simulink model "sim_mobile_robot_trajectory_control_pi"  (R2020b)
settings: Solver=ode1  StartTime=0.0  StopTime=100  FixedStep=0.01  RelTol=1e-3
libraries: pid_lib x2, simulink x2, dspsigops x1
settings Model: Creator=ONLY-GOD  LastModifiedBy=ONLY-GOD

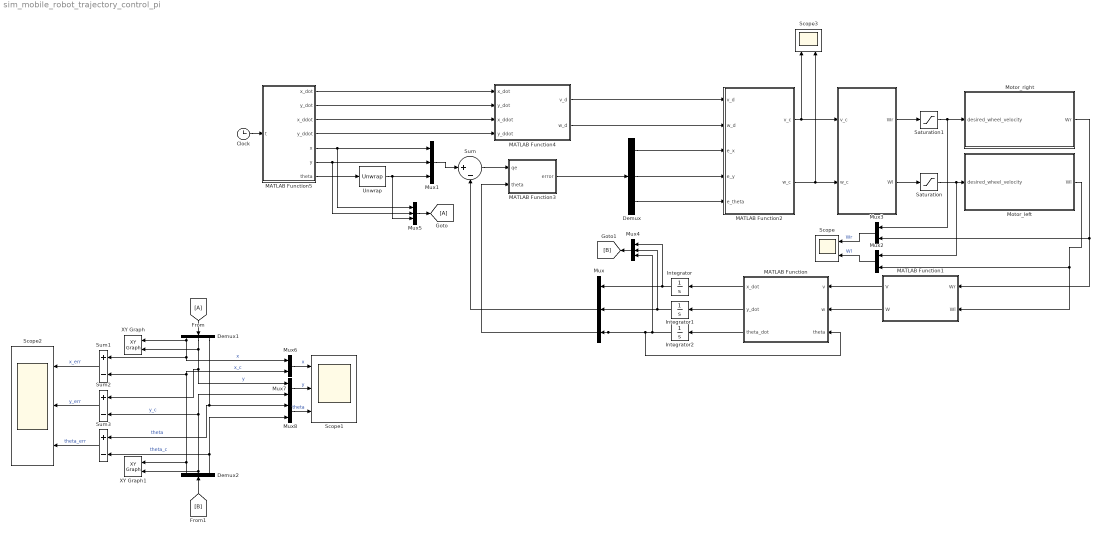
== system sim_mobile_robot_trajectory_control_pi ==
  " " : MATLAB Function  TreatAsAtomicUnit=on
  Clock : Clock
  Demux : Demux  Outputs=3
  Demux1 : Demux  Outputs=3
  Demux2 : Demux  Outputs=3
  Integrator : Integrator
  Integrator1 : Integrator
  Integrator2 : Integrator
  MATLAB Function : MATLAB Function  TreatAsAtomicUnit=on
  MATLAB Function1 : MATLAB Function  TreatAsAtomicUnit=on
  MATLAB Function2 : MATLAB Function  TreatAsAtomicUnit=on
  MATLAB Function3 : MATLAB Function  TreatAsAtomicUnit=on
  MATLAB Function4 : MATLAB Function  TreatAsAtomicUnit=on
  MATLAB Function5 : MATLAB Function  TreatAsAtomicUnit=on
  Motor_left : Subsystem
  Motor_right : Subsystem
  Mux{,1,4..5} (4 alike) : Mux  Inputs=3
  Mux{2..3,6..8} (5 alike) : Mux  Inputs=2
  Saturation : Saturate  UpperLimit=14  LowerLimit=-14
  Saturation1 : Saturate  UpperLimit=14  LowerLimit=-14
  Scope : Scope  NumInputPorts=2
  Scope1 : Scope  NumInputPorts=3
  Scope2 : Scope  NumInputPorts=3
  Scope3 : Scope  NumInputPorts=2
  Sum : Sum  Inputs=|+-
  Sum1 : Sum  Inputs=+-
  Sum2 : Sum  Inputs=+-
  Sum3 : Sum  Inputs=+-
  Unwrap : dspsigops/Unwrap  tol=pi  InputProcessing=Columns as channels (frame based)  running=off
  XY Graph : simulink/Sinks/XY Graph  xmin=-6  xmax=6  ymin=-6  ymax=6  st=-1
  XY Graph1 : simulink/Sinks/XY Graph  xmin=-6  xmax=6  ymin=-6  ymax=6  st=-1
  wires:
  Demux/1 -> MATLAB Function2/3(e_x)
  Demux/2 -> MATLAB Function2/4(e_y)
  Demux/3 -> MATLAB Function2/5(e_theta)
  Sum/1 -> MATLAB Function3/1(qe)
  MATLAB Function3/1(error) -> Demux/1
  MATLAB Function4/1(v_d) -> MATLAB Function2/1(v_d)
  MATLAB Function4/2(w_d) -> MATLAB Function2/2(w_d)
  MATLAB Function2/1(v_c) -> " "/1(v_c), Scope3/1
  MATLAB Function2/2(w_c) -> Scope3/2, " "/2(w_c)
  " "/1(Wr) -> Saturation1/1
  " "/2(Wl) -> Saturation/1
  Motor_right/1(Wr) -> Mux3/2, MATLAB Function1/1(Wr)
  Motor_left/1(Wl) -> Mux2/2, MATLAB Function1/2(Wl)
  MATLAB Function1/1(V) -> MATLAB Function/1(v)
  MATLAB Function1/2(W) -> MATLAB Function/2(w)
  MATLAB Function/3(theta_dot) -> Integrator2/1
  MATLAB Function/1(x_dot) -> Integrator/1
  MATLAB Function/2(y_dot) -> Integrator1/1
  Integrator2/1 -> Mux4/3, MATLAB Function3/2(theta), Mux/3, MATLAB Function/3(theta)
  Integrator/1 -> Mux4/1, Mux/1
  Integrator1/1 -> Mux4/2, Mux/2
  Mux/1 -> Sum/2
  MATLAB Function5/1(x_dot) -> MATLAB Function4/1(x_dot)
  MATLAB Function5/2(y_dot) -> MATLAB Function4/2(y_dot)
  MATLAB Function5/3(x_ddot) -> MATLAB Function4/3(x_ddot)
  MATLAB Function5/4(y_ddot) -> MATLAB Function4/4(y_ddot)
  Clock/1 -> MATLAB Function5/1(t)
  MATLAB Function5/5(x) -> Mux1/1, Mux5/1
  MATLAB Function5/6(y) -> Mux1/2, Mux5/2
  MATLAB Function5/7(theta) -> Unwrap/1
  Mux1/1 -> Sum/1
  Mux3/1 -> Scope/1  "Wr"
  Mux2/1 -> Scope/2  "Wl"
  Mux5/1 -> [A]
  Mux4/1 -> [B]
  [A] -> Demux1/1
  [B] -> Demux2/1
  Demux1/1 -> Mux6/1, Sum1/1, XY Graph/1  "x"
  Demux2/1 -> Mux6/2, Sum1/2, XY Graph1/1  "x_c"
  Demux1/2 -> Sum2/1, Mux7/1, XY Graph/2  "y"
  Demux2/2 -> Mux7/2, Sum2/2, XY Graph1/2  "y_c"
  Demux2/3 -> Mux8/2, Sum3/2  "theta_c"
  Mux6/1 -> Scope1/1  "x"
  Mux7/1 -> Scope1/2  "y"
  Mux8/1 -> Scope1/3  "theta"
  Demux1/3 -> Sum3/1, Mux8/1  "theta"
  Sum1/1 -> Scope2/1  "x_err"
  Sum2/1 -> Scope2/2  "y_err"
  Saturation1/1 -> Mux3/1, Motor_right/1(desired_wheel_velocity)
  Saturation/1 -> Mux2/1, Motor_left/1(desired_wheel_velocity)
  Unwrap/1 -> Mux5/3, Mux1/3
  Sum3/1 -> Scope2/3  "theta_err"

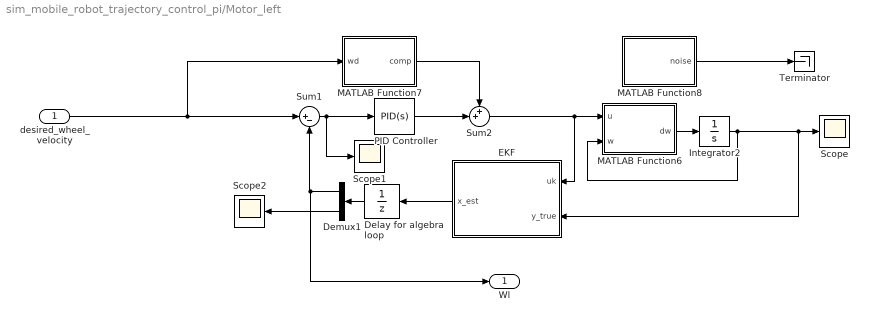
== system sim_mobile_robot_trajectory_control_pi/Motor_left ==
  desired_wheel_velocity : Inport
  Delay for algebra loop : UnitDelay  SampleTime=-1  HasFrameUpgradeWarning=on
  Demux1 : Demux  Outputs=[1,3]
  EKF : MATLAB Function  TreatAsAtomicUnit=on
  Integrator2 : Integrator
  MATLAB Function6 : MATLAB Function  TreatAsAtomicUnit=on
  MATLAB Function7 : MATLAB Function  TreatAsAtomicUnit=on
  MATLAB Function8 : MATLAB Function  TreatAsAtomicUnit=on
  PID Controller : pid_lib/PID Controller  Controller=PID  Form=Parallel  TimeDomain=Continuous-time  UseExternalTs=off  SampleTime=-1  IntegratorMethod=Forward Euler  FilterMethod=Forward Euler  ControllerParametersSource=internal  P=3*(27.65*(-1+2*1.5-2*sqrt(1.5*(1.5-1)))/17.35)  I=3*(27.65*(-1+2*1.5-2*sqrt(1.5*(1.5-1)))/17.35)* 1.5*27.65  D=0  UseFilter=on  N=100  TunerSelectOption=Transfer Function Based (PID Tuner App)  InitialConditionSource=internal  InitialConditionForIntegrator=0  InitialConditionForFilter=0  DifferentiatorICPrevScaledInput=0  ExternalReset=none  TrackingMode=off  Kt=1  LimitOutput=off  SatLimitsSource=internal  UpperSaturationLimit=inf  LowerSaturationLimit=-inf  LinearizeAsGain=on  AntiWindupMode=none  Kb=1  POutMin=[]  POutMax=[]  IOutMin=[]  IOutMax=[]  DOutMin=[]  DOutMax=[]  NOutMin=[]  NOutMax=[]  SumOutMin=[]  SumOutMax=[]  SaturationOutMin=[]  SaturationOutMax=[]  PParamMin=[]  PParamMax=[]  IParamMin=[]  IParamMax=[]  DParamMin=[]  DParamMax=[]  NParamMin=[]  NParamMax=[]  KbParamMin=[]  KbParamMax=[]  KtParamMin=[]  KtParamMax=[]  KbOutMin=[]  KbOutMax=[]  KtOutMin=[]  KtOutMax=[]  IntegratorOutMin=[]  IntegratorOutMax=[]  FilterOutMin=[]  FilterOutMax=[]  SumI1OutMin=[]  SumI1OutMax=[]  SumI2OutMin=[]  SumI2OutMax=[]  SumI3OutMin=[]  SumI3OutMax=[]  SumI4OutMin=[]  SumI4OutMax=[]  SumDOutMin=[]  SumDOutMax=[]  DifferentiatorOutMin=[]  DifferentiatorOutMax=[]  FilterDiffOutCoefMin=[]  FilterDiffOutCoefMax=[]  ReciprocalOutMin=[]  ReciprocalOutMax=[]  SumDenOutMin=[]  SumDenOutMax=[]  SumNumOutMin=[]  SumNumOutMax=[]  DivideOutMin=[]  DivideOutMax=[]  UdiffTsProdOutMin=[]  UdiffTsProdOutMax=[]  NTsProdOutMin=[]  NTsProdOutMax=[]  UintegralTsProdOutMin=[]  UintegralTsProdOutMax=[]  UngainTsProdOutMin=[]  UngainTsProdOutMax=[]  IntegratorContinuousStateAttributes=''  IntegratorStateMustResolveToSignalObject=off  IntegratorRTWStateStorageClass=Auto  FilterContinuousStateAttributes=''  FilterStateMustResolveToSignalObject=off  FilterRTWStateStorageClass=Auto  ParallelPVariant=InternalParameters  IdealPVariant=Disabled  IVariant=InternalParameters  DVariant=InternalParameters  IntegratorVariant=Continuous  SatVariant=Disabled  AWVariant=Passthrough  PCopyVariant=Disabled  TRVariant=Disabled  FdbkBlocksVariant=Forward  IdealPFdbkVariant=Disabled  SatFdbkVariant=Disabled  DerivativeFilterVariant=ContFilter  NVariant=InternalParameters  NCopyVariant=Disabled  FilterICVariant=InternalICsFilter  IntegratorICVariant=InternalICs  ExternalResetVariant=Disabled  TRSumVariant=Passthrough  SumFdbkVariant=Disabled  SumVariant=Sum_PID  TsampFilterVariant=InternalTs  TsampNgainVariant=Passthrough  TsampIntegralVariant=Passthrough  ExternalSaturationOutDataTypeStr=Inherit: Same as second input
  Scope : Scope
  Scope1 : Scope
  Scope2 : Scope
  Sum1 : Sum  Inputs=|+-
  Sum2 : Sum  Inputs=++|
  Terminator : Terminator
  Wl : Outport
  wires:
  Delay for algebra loop/1 -> Demux1/1
  Demux1/1 -> Wl/1, Sum1/2
  Integrator2/1 -> MATLAB Function6/2(w), Scope/1, EKF/2(y_true)
  MATLAB Function7/1(comp) -> Sum2/1
  Demux1/2 -> Scope2/1
  MATLAB Function8/1(noise) -> Terminator/1
  EKF/1(x_est) -> Delay for algebra loop/1
  MATLAB Function6/1(dw) -> Integrator2/1
  PID Controller/1 -> Sum2/2
  Sum1/1 -> PID Controller/1, Scope1/1
  desired_wheel_velocity/1 -> Sum1/1, MATLAB Function7/1(wd)
  Sum2/1 -> MATLAB Function6/1(u), EKF/1(uk)

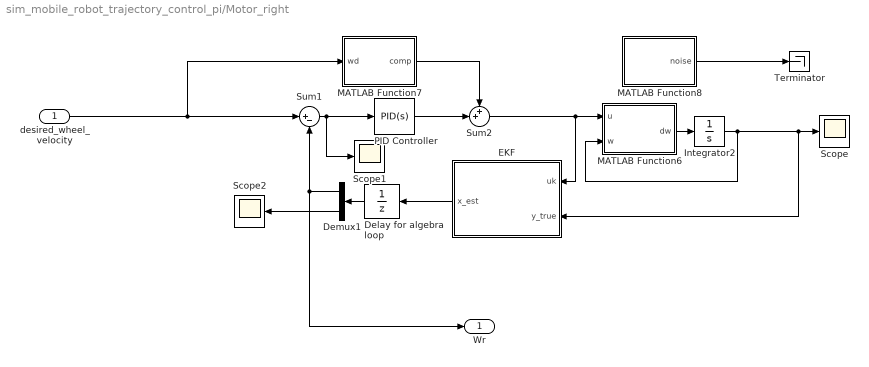
== system sim_mobile_robot_trajectory_control_pi/Motor_right ==
  desired_wheel_velocity : Inport
  Delay for algebra loop : UnitDelay  SampleTime=-1  HasFrameUpgradeWarning=on
  Demux1 : Demux  Outputs=[1,3]
  EKF : MATLAB Function  TreatAsAtomicUnit=on
  Integrator2 : Integrator
  MATLAB Function6 : MATLAB Function  TreatAsAtomicUnit=on
  MATLAB Function7 : MATLAB Function  TreatAsAtomicUnit=on
  MATLAB Function8 : MATLAB Function  TreatAsAtomicUnit=on
  PID Controller : pid_lib/PID Controller  Controller=PID  Form=Parallel  TimeDomain=Continuous-time  UseExternalTs=off  SampleTime=-1  IntegratorMethod=Forward Euler  FilterMethod=Forward Euler  ControllerParametersSource=internal  P=3*(27.65*(-1+2*1.5-2*sqrt(1.5*(1.5-1)))/17.35)  I=3*(27.65*(-1+2*1.5-2*sqrt(1.5*(1.5-1)))/17.35)* 1.5*27.65  D=0  UseFilter=on  N=100  TunerSelectOption=Transfer Function Based (PID Tuner App)  InitialConditionSource=internal  InitialConditionForIntegrator=0  InitialConditionForFilter=0  DifferentiatorICPrevScaledInput=0  ExternalReset=none  TrackingMode=off  Kt=1  LimitOutput=off  SatLimitsSource=internal  UpperSaturationLimit=inf  LowerSaturationLimit=-inf  LinearizeAsGain=on  AntiWindupMode=none  Kb=1  POutMin=[]  POutMax=[]  IOutMin=[]  IOutMax=[]  DOutMin=[]  DOutMax=[]  NOutMin=[]  NOutMax=[]  SumOutMin=[]  SumOutMax=[]  SaturationOutMin=[]  SaturationOutMax=[]  PParamMin=[]  PParamMax=[]  IParamMin=[]  IParamMax=[]  DParamMin=[]  DParamMax=[]  NParamMin=[]  NParamMax=[]  KbParamMin=[]  KbParamMax=[]  KtParamMin=[]  KtParamMax=[]  KbOutMin=[]  KbOutMax=[]  KtOutMin=[]  KtOutMax=[]  IntegratorOutMin=[]  IntegratorOutMax=[]  FilterOutMin=[]  FilterOutMax=[]  SumI1OutMin=[]  SumI1OutMax=[]  SumI2OutMin=[]  SumI2OutMax=[]  SumI3OutMin=[]  SumI3OutMax=[]  SumI4OutMin=[]  SumI4OutMax=[]  SumDOutMin=[]  SumDOutMax=[]  DifferentiatorOutMin=[]  DifferentiatorOutMax=[]  FilterDiffOutCoefMin=[]  FilterDiffOutCoefMax=[]  ReciprocalOutMin=[]  ReciprocalOutMax=[]  SumDenOutMin=[]  SumDenOutMax=[]  SumNumOutMin=[]  SumNumOutMax=[]  DivideOutMin=[]  DivideOutMax=[]  UdiffTsProdOutMin=[]  UdiffTsProdOutMax=[]  NTsProdOutMin=[]  NTsProdOutMax=[]  UintegralTsProdOutMin=[]  UintegralTsProdOutMax=[]  UngainTsProdOutMin=[]  UngainTsProdOutMax=[]  IntegratorContinuousStateAttributes=''  IntegratorStateMustResolveToSignalObject=off  IntegratorRTWStateStorageClass=Auto  FilterContinuousStateAttributes=''  FilterStateMustResolveToSignalObject=off  FilterRTWStateStorageClass=Auto  ParallelPVariant=InternalParameters  IdealPVariant=Disabled  IVariant=InternalParameters  DVariant=InternalParameters  IntegratorVariant=Continuous  SatVariant=Disabled  AWVariant=Passthrough  PCopyVariant=Disabled  TRVariant=Disabled  FdbkBlocksVariant=Forward  IdealPFdbkVariant=Disabled  SatFdbkVariant=Disabled  DerivativeFilterVariant=ContFilter  NVariant=InternalParameters  NCopyVariant=Disabled  FilterICVariant=InternalICsFilter  IntegratorICVariant=InternalICs  ExternalResetVariant=Disabled  TRSumVariant=Passthrough  SumFdbkVariant=Disabled  SumVariant=Sum_PID  TsampFilterVariant=InternalTs  TsampNgainVariant=Passthrough  TsampIntegralVariant=Passthrough  ExternalSaturationOutDataTypeStr=Inherit: Same as second input
  Scope : Scope
  Scope1 : Scope
  Scope2 : Scope
  Sum1 : Sum  Inputs=|+-
  Sum2 : Sum  Inputs=++|
  Terminator : Terminator
  Wr : Outport
  wires:
  Sum2/1 -> MATLAB Function6/1(u), EKF/1(uk)
  desired_wheel_velocity/1 -> MATLAB Function7/1(wd), Sum1/1
  Sum1/1 -> Scope1/1, PID Controller/1
  PID Controller/1 -> Sum2/2
  MATLAB Function6/1(dw) -> Integrator2/1
  EKF/1(x_est) -> Delay for algebra loop/1
  MATLAB Function8/1(noise) -> Terminator/1
  Demux1/2 -> Scope2/1
  MATLAB Function7/1(comp) -> Sum2/1
  Integrator2/1 -> MATLAB Function6/2(w), EKF/2(y_true), Scope/1
  Demux1/1 -> Wr/1, Sum1/2
  Delay for algebra loop/1 -> Demux1/1

== matlab function sim_mobile_robot_trajectory_control_pi/Motor_left/MATLAB Function7 ==
  settings: updateMethod=DISCRETE
  data: wd input; comp output
function comp = fcn(wd)

b = 17.35 + rand; c = 5.63 + 0.3*rand;
comp = c/b*sign(wd);

== matlab function sim_mobile_robot_trajectory_control_pi/Motor_left/MATLAB Function8 ==
  data: noise output
function noise = fcn

noise = 0.1*randn;

== matlab function sim_mobile_robot_trajectory_control_pi/MATLAB Function1 ==
  data: Wr input; V output; Wl input; W output
function [V,W]= fcn(Wr,Wl)
r = 0.07;      %wheel radius
b = 0.22;      %length from wheel to wheel

V = r*(Wr/2) + r*(Wl/2);
W = r*(Wr/b) - r*(Wl/b);

== matlab function sim_mobile_robot_trajectory_control_pi/MATLAB Function5 ==
  data: x_dot output; y_dot output; x_ddot output; y_ddot output; x output; t input; y output; theta output
function [x_dot,y_dot,x_ddot,y_ddot,x,y,theta] = ref(t)

f = 2*pi*0.01;
r = 4;

x = r*cos(f*t);
y = r*sin(f*t);

x_dot = -r*f*sin(f*t);
y_dot = r*f*cos(f*t);

theta = atan2(y_dot,x_dot);

x_ddot = -r*f^2*cos(f*t);
y_ddot = -r*f^2*sin(f*t);

== matlab function sim_mobile_robot_trajectory_control_pi/Motor_left/EKF ==
  settings: updateMethod=DISCRETE
  data: uk input; y_true input; x_est output
function x_est = EKF(uk,y_true)
Ts=0.01;
persistent x_est_p P Qd_est R_est Qc_est;
if isempty(x_est_p)
    
    x_est_p=[2;13;25;1];
    P=2*eye(4);
    Qc_est=1e-5*diag([10,25,25,1]);
    Qd_est=Qc_est*Ts;
    R_est=0.02;
end
c=[1 0 0 0];D=0;Ck=c;Dk=D;
%Comput Kalman Gain and update predicted value
Wk=P*Ck'/(Ck*P*Ck'+R_est);
y_est=Ck*x_est_p+Dk*uk;
x=x_est_p+Wk.*(y_true-y_est);
%Compute prediction at next time step
x_est=x+Ts*[-x(2)*x(1)+uk*x(3)-x(4)*sign(x(1));0;0;0];
%Update error covariance matrices
P=P-Wk*Ck*P;
%Define Ak
Ak=eye(4)+Ts*[-x(2) -x(1) uk -sign(x(1));0 0 0 0;0 0 0 0;0 0 0 0]; % jacobian
P=Ak*P*Ak'+Qd_est;
x_est_p=x_est;

== matlab function sim_mobile_robot_trajectory_control_pi/  ==
  data: v_c input; Wr output; w_c input; Wl output
function [Wr, Wl] = M_inv(v_c, w_c)
r = 0.07;      %wheel radius
b = 0.22;      %length from wheel to wheel

Wr = ((2*v_c)+(w_c*b))/(2*r);
Wl = ((2*v_c)-(w_c*b))/(2*r);

== matlab function sim_mobile_robot_trajectory_control_pi/MATLAB Function ==
  data: v input; x_dot output; w input; y_dot output; theta_dot output; theta input
function [x_dot,y_dot,theta_dot]= kinematic(v,w,theta)
x_dot = v*cos(theta);
y_dot = v*sin(theta);
theta_dot = w;

== matlab function sim_mobile_robot_trajectory_control_pi/MATLAB Function2 ==
  data: v_d input; v_c output; w_d input; e_x input; e_y input; e_theta input; w_c output
function [v_c,w_c] =  bckstep(v_d, w_d, e_x, e_y, e_theta)            

% control gain
k1 = 1;
k2 = 20 ;
k3 = 1 ;

v_c = k1*e_x + v_d*cos(e_theta);
w_c = w_d + k2*v_d*e_y + k3*v_d*sin(e_theta);

== matlab function sim_mobile_robot_trajectory_control_pi/MATLAB Function3 ==
  data: qe input; error output; theta input
function error = rotation(qe,theta)

T = [cos(theta) , sin(theta) , 0 ;
    -sin(theta) , cos(theta) , 0 ;
         0      ,     0      , 1 ];
     
error = T*qe;

== matlab function sim_mobile_robot_trajectory_control_pi/MATLAB Function4 ==
  data: x_dot input; v_d output; w_d output; y_dot input; x_ddot input; y_ddot input
function [v_d,w_d] = fcn(x_dot,y_dot,x_ddot,y_ddot)

v_d = sqrt(x_dot^2 + y_dot^2);
w_d = ((x_dot*y_ddot)-(y_dot*x_ddot))/((x_dot^2 + y_dot^2));

== matlab function sim_mobile_robot_trajectory_control_pi/Motor_left/MATLAB Function6 ==
  settings: updateMethod=DISCRETE
  data: u input; dw output; w input
function dw = dcmotor(u,w)

a = 27.65; b = 17.35; c = 5.63;
dw = -a*w+b*u-c*sign(w) + 1e-4*randn;

== matlab function sim_mobile_robot_trajectory_control_pi/Motor_right/EKF ==
  settings: updateMethod=DISCRETE
  data: uk input; y_true input; x_est output
function x_est = EKF(uk,y_true)
Ts=0.01;
persistent x_est_p P Qd_est R_est Qc_est;
if isempty(x_est_p)
    
    x_est_p=[2;13;25;1];
    P=2*eye(4);
    Qc_est=1e-5*diag([10,25,25,1]);
    Qd_est=Qc_est*Ts;
    R_est=0.02;
end
c=[1 0 0 0];D=0;Ck=c;Dk=D;
%Comput Kalman Gain and update predicted value
Wk=P*Ck'/(Ck*P*Ck'+R_est);
y_est=Ck*x_est_p+Dk*uk;
x=x_est_p+Wk.*(y_true-y_est);
%Compute prediction at next time step
x_est=x+Ts*[-x(2)*x(1)+uk*x(3)-x(4)*sign(x(1));0;0;0];
%Update error covariance matrices
P=P-Wk*Ck*P;
%Define Ak
Ak=eye(4)+Ts*[-x(2) -x(1) uk -sign(x(1));0 0 0 0;0 0 0 0;0 0 0 0]; % jacobian
P=Ak*P*Ak'+Qd_est;
x_est_p=x_est;

== matlab function sim_mobile_robot_trajectory_control_pi/Motor_right/MATLAB Function6 ==
  settings: updateMethod=DISCRETE
  data: u input; dw output; w input
function dw = dcmotor(u,w)

a = 27.65; b = 17.35; c = 5.63;
dw = -a*w+b*u-c*sign(w) + 1e-4*randn;

== matlab function sim_mobile_robot_trajectory_control_pi/Motor_right/MATLAB Function7 ==
  settings: updateMethod=DISCRETE
  data: wd input; comp output
function comp = fcn(wd)

b = 17.35 + rand; c = 5.63 + 0.3*rand;
comp = c/b*sign(wd);

== matlab function sim_mobile_robot_trajectory_control_pi/Motor_right/MATLAB Function8 ==
  data: noise output
function noise = fcn

noise = 0.1*randn;
